simulink model "Example_Model"  (R2018a)
settings: Solver=ode15s  StartTime=0.0  StopTime=20  RelTol=1e-10  AbsTol=1e-13
settings Model: SimulationMode=accelerator  Creator=jnicholson  LastModifiedBy=jnicholson

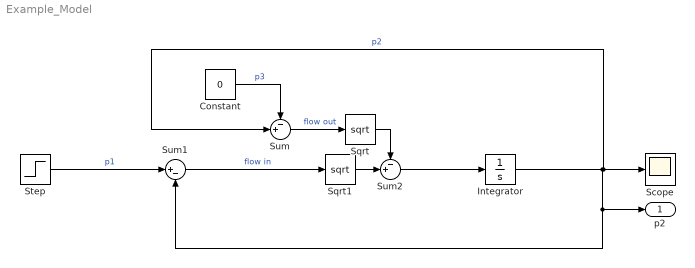
== system Example_Model ==
  Constant : Constant  Value=0
  Integrator : Integrator  ZeroCross=off  ContinuousStateAttributes='p2'
  Scope : Scope
  Sqrt : Sqrt  SaturateOnIntegerOverflow=on
  Sqrt1 : Sqrt  SaturateOnIntegerOverflow=on
  Step : Step  Before=1  After=10  SampleTime=0
  Sum : Sum  Inputs=-+|
  Sum1 : Sum  Inputs=|+-
  Sum2 : Sum  Inputs=-+|
  p2 : Outport
  wires:
  Step/1 -> Sum1/1  "p1"
  Integrator/1 -> p2/1, Sum1/2, Sum/2, Scope/1  "p2"
  Sum1/1 -> Sqrt1/1  "flow in"
  Constant/1 -> Sum/1  "p3"
  Sum/1 -> Sqrt/1  "flow out"
  Sum2/1 -> Integrator/1
  Sqrt/1 -> Sum2/1
  Sqrt1/1 -> Sum2/2
